simulink model "SOC_Estimation"  (R2022b)
settings: configuration reference "BMS_Sw_CodeGenConfig" (kept outside this file)
undefined symbols (not defined in the file): battery_sli_rtmsupport, BatteryNN, BMS_State_Enum, C1_mat, c_sqrt, DiscIntNeverNeededParam, dV0_mat, gcbh, n, Np_Module, Ns_Module, NumModules, SOCInit, Wc, Wm, x0
libraries: simulink x1
(part 2 of 2)

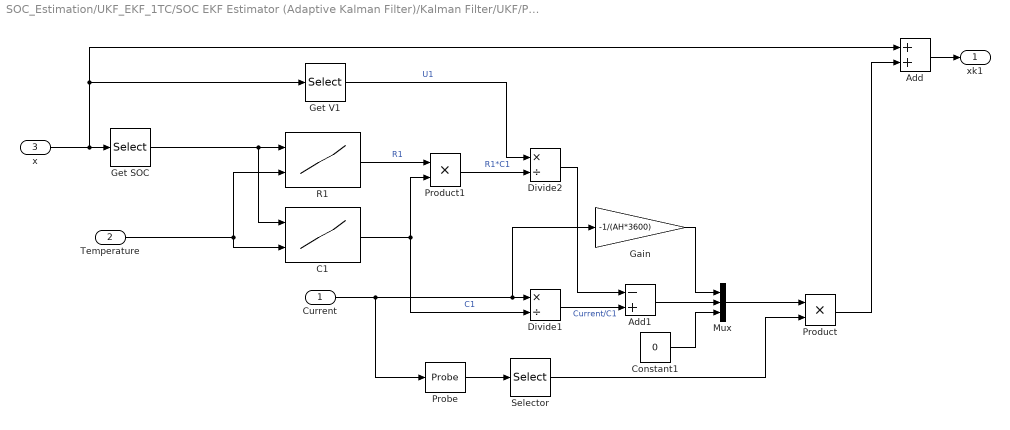
== system SOC_Estimation/UKF_EKF_1TC/SOC EKF Estimator (Adaptive Kalman Filter)/Kalman Filter/UKF/Prediction/State function/State function ==
  Current : Inport
  Temperature : Inport  Port=2
  x : Inport  Port=3
  Add : Sum
  Add1 : Sum  Inputs=-+
  C1 : Lookup_n-D  BreakpointsForDimension1=SOC_vec  BreakpointsForDimension2=T_vec  BeginIndexSearchUsingPreviousIndexResult=on  Table=C1_mat  ExtrapMethod=Clip  InternalRulePriority=Speed  RndMeth=Simplest
      settings: InputPortMap=u0,u1
  Constant1 : Constant  Value=0
  Divide1 : Product  Inputs=*/
  Divide2 : Product  Inputs=*/
  Gain : Gain  Gain=-1/(AH*3600)
  Get SOC : Selector  InputPortWidth=3  IndexOptions=Index vector (dialog)  Indices=1  OutputSizes=1
  Get V1 : Selector  InputPortWidth=3  IndexOptions=Index vector (dialog)  Indices=2  OutputSizes=1
  Mux : Mux  Inputs=3
  Probe : Probe  ProbeWidth=off  ProbeComplexSignal=off
  Product : Product  OutDataTypeStr=single
  Product1 : Product
  R1 : Lookup_n-D  BreakpointsForDimension1=SOC_vec  BreakpointsForDimension2=T_vec  BeginIndexSearchUsingPreviousIndexResult=on  Table=R1_mat  ExtrapMethod=Clip  InternalRulePriority=Speed  RndMeth=Simplest
      settings: InputPortMap=u0,u1
  Selector : Selector  InputPortWidth=2  IndexOptions=Index vector (dialog)  Indices=1  OutputSizes=1
  xk1 : Outport
  wires:
  Probe/1 -> Selector/1
  Constant1/1 -> Mux/3
  Temperature/1 -> R1/2, C1/2
  x/1 -> Get SOC/1, Get V1/1, Add/1
  Product/1 -> Add/2
  Add1/1 -> Mux/2
  Add/1 -> xk1/1
  Divide2/1 -> Add1/1
  Mux/1 -> Product/1
  Selector/1 -> Product/2
  Current/1 -> Gain/1, Divide1/1, Probe/1
  C1/1 -> Divide1/2, Product1/2  "C1"
  Get V1/1 -> Divide2/1  "U1"
  R1/1 -> Product1/1  "R1"
  Get SOC/1 -> R1/1, C1/1
  Product1/1 -> Divide2/2  "R1*C1"
  Divide1/1 -> Add1/2  "Current/C1"
  Gain/1 -> Mux/1

== matlab function SOC_Estimation/UKF_EKF_1TC/SOC EKF Estimator (Adaptive Kalman Filter)/Kalman Filter/UKF/Correction/updatePk ==
  data: U input; Pk1_k input; Pk1_k1 output; m parameter
function Pk1_k1=updatePk(U,Pk1_k,m)
% Covariance update
%Inputs:
%   U     : U=K*Py'
%   Pk1_k : Covariance at last sample
%   m     : Number of measurements
%Output:
%   Pk1_k1: Updated covariance matrix at (k+1)

% Iterate from 1 to number of measurements

Pk1_k1=battery.control.estimators.CovarianceUpdate(U,Pk1_k,m);

== matlab function SOC_Estimation/UKF_EKF_1TC/SOC EKF Estimator (Adaptive Kalman Filter)/Kalman Filter/UKF/Prediction/updatePx ==
  data: X input; x input; Pk1k output; X1 output; Wc parameter; Q parameter
function [Pk1k,X1]=updateP(X,x, Wc, Q)
% Transformed square root of covariance matrix
%Inputs:
%    X  : Sigma points
%    x  : xhat(k+1|k)
%    Wc : Covariance weight 
%    Q  : Covariance of the process noise
%Outputs:
%    Pk1_k: transformed square root of covariance
%    X1: transformed deviations

[Pk1k,X1]=battery.control.estimators.UnscentedTransformationUpdate(X,x, Wc, Q);

== matlab function SOC_Estimation/UKF_EKF_1TC/SOC EKF Estimator (Adaptive Kalman Filter)/Kalman Filter/UKF/Prediction/updatePy ==
  data: Y input; y input; Py output; Y1 output; Wc parameter; R parameter
function [Py,Y1]=updatePy(Y,y, Wc, R)
% Transformed square root of covariance matrix
%Inputs:
%    Y  : Sigma points
%    y  : yhat(k+1|k)
%    Wc : Covariance weight 
%    R  : Covariance of the measurement noise
%Outputs:
%    Py: transformed square root of covariance
%    Y1: transformed deviations

[Py,Y1]=battery.control.estimators.UnscentedTransformationUpdate(Y,y, Wc, R);
